simulink model "gainControl"  (R2023a)
settings: Solver=VariableStepAuto  StartTime=0.0  StopTime=tStop  MaxStep=tStepSize  RelTol=1e-3
undefined symbols (not defined in the file): tDelay
settings Model: Creator=athmajanvivekananthan  LastModifiedBy=athmajanvivekananthan

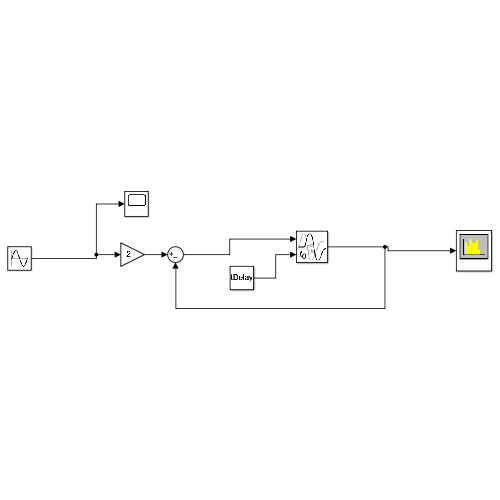
[thumbnail: Simulink's stored preview of the top-level diagram]
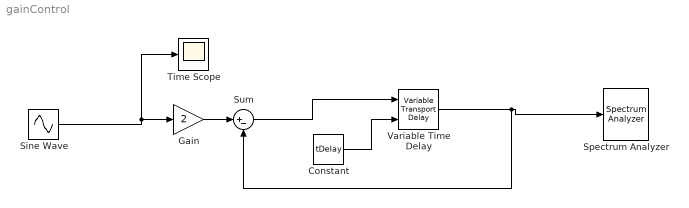
== system gainControl ==
  Constant : Constant  Value=tDelay
  Gain : Gain  Gain=2
  Sine Wave : Sin  SampleTime=0
  Spectrum Analyzer : SpectrumAnalyzer  WindowPosition=[356.000000,241.000000,800.000000,500.000000,]  ScopeFrameLocation=window  ColorLimits=[-80 20]
  Sum : Sum  Inputs=|+-
  Time Scope : Scope
  Variable Time Delay : VariableTransportDelay  MaximumDelay=100
  wires:
  Constant/1 -> Variable Time Delay/2
  Sine Wave/1 -> Gain/1, Time Scope/1
  Variable Time Delay/1 -> Spectrum Analyzer/1, Sum/2
  Gain/1 -> Sum/1
  Sum/1 -> Variable Time Delay/1
